simulink model "Control_ABB"  (R2020b)
settings: Solver=FixedStepAuto  StartTime=0.0  StopTime=20  FixedStep=0.001  RelTol=1e-3
undefined symbols (not defined in the file): X, Y, Z
libraries: sm_lib x57, nesl_utility x13, simulink x2
(part 3 of 3)

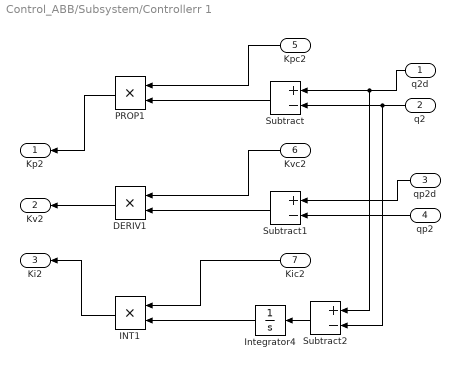
== system Control_ABB/Subsystem/Controllerr 1 ==
  q2d : Inport
  q2 : Inport  Port=2
  qp2d : Inport  Port=3
  qp2 : Inport  Port=4
  Kpc2 : Inport  Port=5
  Kvc2 : Inport  Port=6
  Kic2 : Inport  Port=7
  DERIV1 : Product
  INT1 : Product
  Integrator4 : Integrator
  PROP1 : Product
  Subtract : Sum  Inputs=+-
  Subtract1 : Sum  Inputs=+-
  Subtract2 : Sum  Inputs=+-
  Kp2 : Outport  VectorParamsAs1DForOutWhenUnconnected=off
  Kv2 : Outport  Port=2  VectorParamsAs1DForOutWhenUnconnected=off
  Ki2 : Outport  Port=3  VectorParamsAs1DForOutWhenUnconnected=off
  wires:
  q2/1 -> Subtract2/2, Subtract/2
  qp2/1 -> Subtract1/2
  INT1/1 -> Ki2/1
  Kvc2/1 -> DERIV1/1
  qp2d/1 -> Subtract1/1
  Subtract1/1 -> DERIV1/2
  q2d/1 -> Subtract2/1, Subtract/1
  Kic2/1 -> INT1/1
  DERIV1/1 -> Kv2/1
  Subtract/1 -> PROP1/2
  PROP1/1 -> Kp2/1
  Subtract2/1 -> Integrator4/1
  Integrator4/1 -> INT1/2
  Kpc2/1 -> PROP1/1

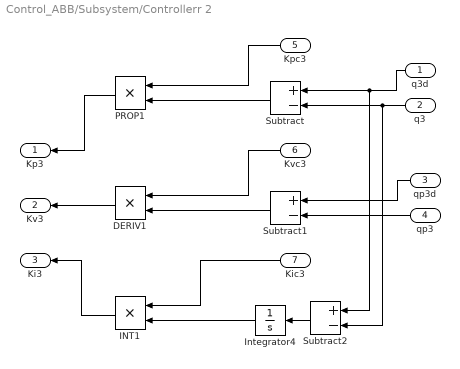
== system Control_ABB/Subsystem/Controllerr 2 ==
  q3d : Inport
  q3 : Inport  Port=2
  qp3d : Inport  Port=3
  qp3 : Inport  Port=4
  Kpc3 : Inport  Port=5
  Kvc3 : Inport  Port=6
  Kic3 : Inport  Port=7
  DERIV1 : Product
  INT1 : Product
  Integrator4 : Integrator
  PROP1 : Product
  Subtract : Sum  Inputs=+-
  Subtract1 : Sum  Inputs=+-
  Subtract2 : Sum  Inputs=+-
  Kp3 : Outport  VectorParamsAs1DForOutWhenUnconnected=off
  Kv3 : Outport  Port=2  VectorParamsAs1DForOutWhenUnconnected=off
  Ki3 : Outport  Port=3  VectorParamsAs1DForOutWhenUnconnected=off
  wires:
  Kpc3/1 -> PROP1/1
  Integrator4/1 -> INT1/2
  Subtract2/1 -> Integrator4/1
  PROP1/1 -> Kp3/1
  Subtract/1 -> PROP1/2
  DERIV1/1 -> Kv3/1
  Kic3/1 -> INT1/1
  q3d/1 -> Subtract/1, Subtract2/1
  Subtract1/1 -> DERIV1/2
  qp3d/1 -> Subtract1/1
  Kvc3/1 -> DERIV1/1
  INT1/1 -> Ki3/1
  qp3/1 -> Subtract1/2
  q3/1 -> Subtract/2, Subtract2/2

== matlab function Control_ABB/Subsystem/COMPENSADOR DE GRAVEDAD ==
  data: q2 input; q3 input; gc output; m2 input; I2 input; m3 input; I3 input; lc2 input; L2 input; lc3 input; L3 input
function gc = g(q2, q3, m2, I2, m3, I3, lc2, L2, lc3, L3)

% Parametros del robot
%m2=23.902; m3=3.88;
%L2=0.45; L3=0.45; lc2=0.091;lc3=0.0229;
%I2=1.266; I3=0.093;

g2c=(m2*lc2+m3*L2)*9.8*sin(q2)+m3*lc3*9.8*sin(q2+q3);
g3c=m3*lc3*9.8*sin(q2+q3);
G=[g2c g3c]';

gc = [g2c;g3c];
